simulink subsystem "LegoMotor"  (R2020a)
settings: Solver=VariableStepAuto  StartTime=0.0  StopTime=10.0  RelTol=1e-3
model mask{ResetMode=No reset}
  mask prompts: ResetMode "Reset Mode"
libraries: simulink_extras x1
Description:
  | Simulates an EV3 Large Servo Motor.
  | The input is motor power, equivalent -100-100 scale that the EV3 Motor block uses.
  | There are two encoder outputs:
  | Encoder Position outputs the cumulative position, like the default EV3 Encoder Block
  | Encoder Change outputs the change in position each sample, equivalent to the EV3 Encoder Block when set to "Reset every sample"
settings Model: Creator=Thomas  LastModifiedBy=abatra2

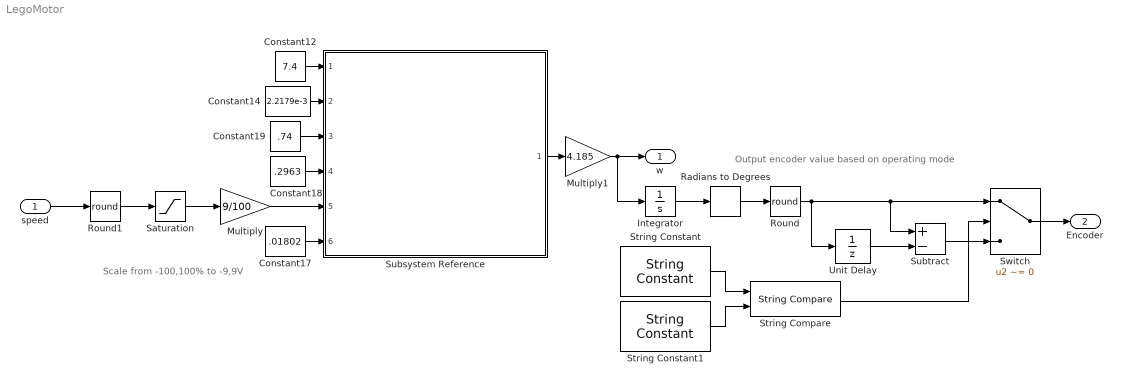
== system LegoMotor ==
  note: Output encoder value based on operating mode
  note: Scale from -100,100% to -9,9V
  speed : Inport
  Constant12 : Constant  Value=7.4
  Constant14 : Constant  Value=2.2179e-3
  Constant17 : Constant  Value=.01802
  Constant18 : Constant  Value=.2963
  Constant19 : Constant  Value=.74
  Integrator : Integrator
  Multiply : Gain  Gain=9/100
  Multiply1 : Gain  Gain=4.185
  Radians to Degrees : simulink_extras/Transformations/Radians to Degrees
  Round : Rounding  Operator=round
  Round1 : Rounding  Operator=round
  Saturation : Saturate  UpperLimit=100  LowerLimit=-100
  String Compare : StringCompare
  String Constant : StringConstant  String=ResetMode
  String Constant1 : StringConstant  String="\"No reset\""
  Subsystem Reference : Subsystem  ReferencedSubsystem=DCMotor
  Subtract : Sum  Inputs=+-
  Switch : Switch  Criteria=u2 ~= 0
  Unit Delay : UnitDelay  SampleTime=-1  HasFrameUpgradeWarning=on
  w : Outport
  Encoder : Outport  Port=2
  wires:
  Constant12/1 -> Subsystem Reference/1
  Constant14/1 -> Subsystem Reference/2
  Constant19/1 -> Subsystem Reference/3
  Constant18/1 -> Subsystem Reference/4
  Constant17/1 -> Subsystem Reference/6
  Multiply/1 -> Subsystem Reference/5
  Round/1 -> Unit Delay/1, Subtract/1, Switch/1
  Unit Delay/1 -> Subtract/2
  Subsystem Reference/1 -> Multiply1/1
  Integrator/1 -> Radians to Degrees/1
  Radians to Degrees/1 -> Round/1
  String Constant/1 -> String Compare/1
  String Constant1/1 -> String Compare/2
  String Compare/1 -> Switch/2
  Switch/1 -> Encoder/1
  Subtract/1 -> Switch/3
  speed/1 -> Round1/1
  Multiply1/1 -> Integrator/1, w/1
  Round1/1 -> Saturation/1
  Saturation/1 -> Multiply/1
